simulink model "Test_Digital_Output_Simple"  (R2020b)
settings: Solver=FixedStepAuto  StartTime=0.0  StopTime=Inf  FixedStep=0.1  RelTol=1e-3
libraries: sldrtlib x1
settings Model: Creator=AVS  LastModifiedBy=AVS
settings OptimizationCC: DefaultParameterBehavior=Inlined  EnhancedBackFolding=on  PassReuseOutputArgsAs=Individual arguments  ZeroExternalMemoryAtStartup=off  ZeroInternalMemoryAtStartup=off  OptimizeBlockOrder=speed  DifferentSizesBufferReuse=on  OptimizationCustomize=off  EfficientTunableParamExpr=on
settings DebuggingCC: ParameterTunabilityLossMsg=error
settings SFSimCC: MATLABDynamicMemAlloc=off
settings RTWCC: Description=Embedded Coder  SystemTargetFile=ert.tlc  TemplateMakefile=ert_default_tmf
settings CodeAppCC: ForceParamTrailComments=on  IgnoreCustomStorageClasses=off  OperatorAnnotations=on  SimulinkDataObjDesc=on  SFDataObjDesc=on  InsertBlockDesc=on
settings ERTTargetCC: TargetLangStandard=C99 (ISO)  GenerateSampleERTMain=on  InlinedParameterPlacement=NonHierarchical  ERTCustomFileTemplate=example_file_process.tlc

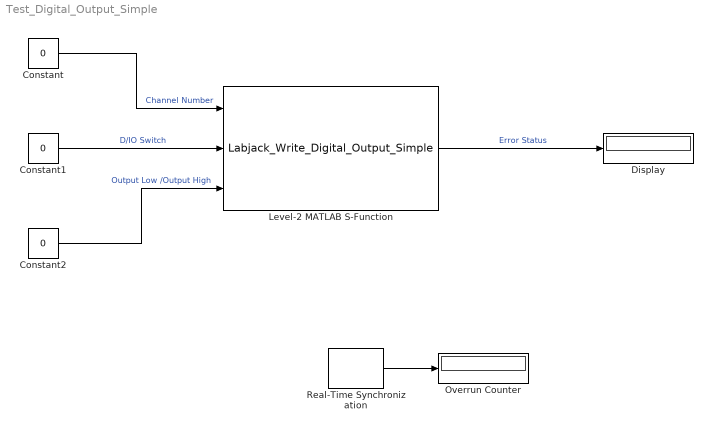
== system Test_Digital_Output_Simple ==
  Constant : Constant  Value=0
  Constant1 : Constant  Value=0
  Constant2 : Constant  Value=0
  Display : Display
  Level-2 MATLAB S-Function : M-S-Function  FunctionName=Labjack_Write_Digital_Output_Simple
  Overrun Counter : Display
  Real-Time Synchronization : sldrtlib/Real-Time Synchronization  SampleTime=0.1  MaxMissedTicks=100  ShowMissedTicks=on  YieldWhenWaiting=off
  wires:
  Level-2 MATLAB S-Function/1 -> Display/1  "Error Status"
  Constant/1 -> Level-2 MATLAB S-Function/1  "Channel Number"
  Real-Time Synchronization/1 -> Overrun Counter/1
  Constant1/1 -> Level-2 MATLAB S-Function/2  "D/IO Switch"
  Constant2/1 -> Level-2 MATLAB S-Function/3  "Output Low /Output High"
